simulink subsystem "differential_decoder"  (R2020a)
settings: Solver=VariableStepAuto  StartTime=0.0  StopTime=10.0  RelTol=1e-3
settings Model: Creator=upattacini  LastModifiedBy=upattacini

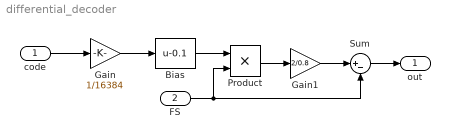
== system differential_decoder ==
  code : Inport
  FS : Inport  Port=2
  Bias : Bias  Bias=-0.1
  Gain : Gain  Gain=1/16384
  Gain1 : Gain  Gain=2/0.8
  Product : Product
  Sum : Sum  Inputs=|+-
  out : Outport
  wires:
  Product/1 -> Gain1/1
  Bias/1 -> Product/1
  Gain1/1 -> Sum/1
  code/1 -> Gain/1
  Gain/1 -> Bias/1
  FS/1 -> Sum/2, Product/2
  Sum/1 -> out/1
